simulink model "Vending_State_Machine"  (R2025b)
settings: Solver=ode45  StartTime=0.0  StopTime=inf  RelTol=1e-3
(part 2 of 2)

== stateflow chart Vending_State_Machine/Chart ==
  state ?
    state VendingMachine
      state MoneyManager
        (history)
        state StockManage
        state Idle
        state Accumulation
        Idle -> Accumulation [order 1] : [InsertCoin==1]
            | {TC(1)=TC(1)+1;TC(2)=TC(2)+1;}
        Accumulation -> Accumulation [order 1] : [InsertCoin==1]
            | {TC(1)=TC(1)+1;TC(2)=TC(2)+1}
        (default) -> Idle
        Accumulation -> Idle [order 4] : [TC(1)==0]
        Accumulation -> StockManage [order 3] : [F>0]{f=F;inStock=2;}
        Idle -> Accumulation [order 2] : [InsertCoin==2]
            | {TC(1)=TC(1)+2;TC(3)=TC(3)+1;}
        (junction 137) -> Accumulation [order 1] : [TC(1)>0]
        StockManage -> (junction 137) : [inStock==1]
        (junction 137) -> Idle [order 2] : [TC(1)==0]
        Accumulation -> Accumulation [order 2] : [InsertCoin==2]
            | {TC(1)=TC(1)+2;TC(3)=TC(3)+1}
      state StockManager
        state Dispenceing
          state Drink [parallel]
            settings: executionOrder=1
            state Despencing
              en,du:
              y=elapsed(sec);
              if y<=2
              motor(f)=1;
              else
              TS(f)=TS(f)-1;
              motor(f)=0;
              y=0;
              end
            state Complete
            (default) -> ?.VendingMachine.StockManager.Dispenceing.Drink.Despencing
            ?.VendingMachine.StockManager.Dispenceing.Drink.Despencing -> ?.VendingMachine.StockManager.Dispenceing.Drink.Complete : [motor(f)==0]
          state Money [parallel]
            settings: executionOrder=2
            state Checking
              en:
              if TC(1)>0
              if TC(1)>1&&TC(3)>=1
              coinDispenser(2)=1;
              else
              if TC(2)>=1
              coinDispenser(1)=1;
              else
              TC(1)=0;
              end
              end
              end
            state Despencing
              en,du:
              y=elapsed(msec);
              if y>=5
              if coinDispenser(2)==1
              TC(3)=TC(3)-1;
              TC(1)=TC(1)-2;
              coinDispenser(2)=0;
              else
              if coinDispenser(1)==1
              TC(2)=TC(2)-1;
              TC(1)=TC(1)-1;
              coinDispenser(1)=0;
              end
              end
              end
            state Complete
            (default) -> ?.VendingMachine.StockManager.Dispenceing.Money.Checking
            ?.VendingMachine.StockManager.Dispenceing.Money.Despencing -> ?.VendingMachine.StockManager.Dispenceing.Money.Checking : [coinDispenser==[0,0]]
            ?.VendingMachine.StockManager.Dispenceing.Money.Checking -> ?.VendingMachine.StockManager.Dispenceing.Money.Despencing [order 1] : [coinDispenser(1)==1||coinDispenser(2)==1]
            ?.VendingMachine.StockManager.Dispenceing.Money.Checking -> ?.VendingMachine.StockManager.Dispenceing.Money.Complete [order 2] : [TC(1)==0]
        state CheckStock
        state checkingTotalStock
          en:
          if TS==[0,0,0,0,0]
          inStock=0;
          else
          inStock=1;
          end
        (default) -> CheckStock
        CheckStock -> Dispenceing [order 1] : [TS(f)>0]{TC(1)=TC(1)-1;despence=1;}
        CheckStock -> checkingTotalStock [order 2] : [TS(f)==0]
        Dispenceing -> checkingTotalStock : [motor(f)==0&&TC(1)==0]
      state Lock
      state DespencingChange
        state Checking
          en:
          if TC(1)>0
          if TC(1)>1&&TC(3)>=1
          coinDispenser(2)=1;
          else
          if TC(2)>=1
          coinDispenser(1)=1;
          else
          TC(1)=0
          end
          end
          end
        state Despencing
          en,du:
          y=elapsed(msec);
          if y>=5
          if coinDispenser(2)==1
          TC(3)=TC(3)-1;
          coinDispenser(2)=0;
          TC(1)=TC(1)-2
          else
          if coinDispenser(1)==1
          TC(2)=TC(2)-1;
          coinDispenser(1)=0;
          TC(1)=TC(1)-1;
          end
          end
          end
        state Complete
        (default) -> ?.VendingMachine.DespencingChange.Checking
        ?.VendingMachine.DespencingChange.Despencing -> ?.VendingMachine.DespencingChange.Checking : [coinDispenser==[0,0]]
        ?.VendingMachine.DespencingChange.Checking -> ?.VendingMachine.DespencingChange.Despencing [order 2] : [coinDispenser(1)==1||coinDispenser(2)==1]
        ?.VendingMachine.DespencingChange.Checking -> ?.VendingMachine.DespencingChange.Complete [order 1] : [TC(1)==0]
      (default) -> MoneyManager
      MoneyManager -> StockManager [order 2] : [inStock==2]{despence=0}
      StockManager -> MoneyManager [order 1] : [inStock==1]
      Lock -> MoneyManager : [Restock==1]
          | {inStock=1;TS=[5,5,5,5,5];}
      (junction 133) -> MoneyManager [order 1] : [inStock==1]
      MoneyManager -> DespencingChange [order 1] : [Cancel==1]
      StockManager -> (junction 129) [order 2] : [inStock==0]
      (junction 129) -> Lock [order 2] : [TC(1)==0]
      (junction 129) -> DespencingChange [order 1] : [TC(1)>0]
      DespencingChange -> (junction 133) : [TC(1)==0]
      (junction 133) -> Lock [order 2] : [inStock==0]
    state Plot
      en, du:
    (default) -> VendingMachine
  data: y local =0; Cancel input; InsertCoin input; Restock input; F input; motor output =[0,0,0,0,0]; despence local =0; TS output =[5,5,5,5,5]; TC output =[0,0,0]; f local =0; inStock output =1; coinDispenser output =[0,0]
